simulink model "MPC_implemented_constrained"  (R2023b)
settings: Solver=VariableStepAuto  StartTime=0.0  StopTime=15  RelTol=1e-3
values from neighbouring files (symbols this model uses):
  E = F    [constr_matrix.m]
  F = [F , F1]    [constr_matrix.m]
  FF = F    [constr_matrix.m]
  G = [G , G1]    [constr_matrix.m]
  Gamma = CZ*Gamma    [constr_matrix.m]    (also in mpc_without_constr.m)
  Psi = CZ*Psi    [constr_matrix.m]    (also in mpc_without_constr.m)
  Q = kron(eye(Hp),Qi)    [constr_matrix.m]    (also in lqr_obs.m = [10 0 0 0; mpc_without_constr.m)
  R = kron(eye(Hu),Ri)    [constr_matrix.m]    (also in lqr_obs.m = 1; mpc_without_constr.m)
  T = zeros(l*Hp,m)    [constr_matrix.m]    (also in mpc_without_constr.m)
  TH = CZ*TH    [constr_matrix.m]    (also in mpc_without_constr.m)
  ts = 2e-2    (= 0.02)    [script_mpc.m]
  Ts = 0.02    [system_configuration.m]
  u_nom = 0    [system_configuration.m]
  y_nom = [0 0]    [system_configuration.m]
undefined symbols (not defined in the file or in its folder): a_max, Hu, T_regime, Td, Tsalita
libraries: cstblocks x6
settings Model: Creator=aniello  LastModifiedBy=aniello

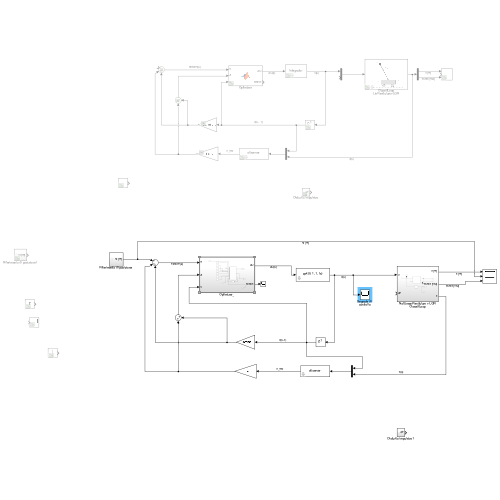
[thumbnail: Simulink's stored preview of the top-level diagram]
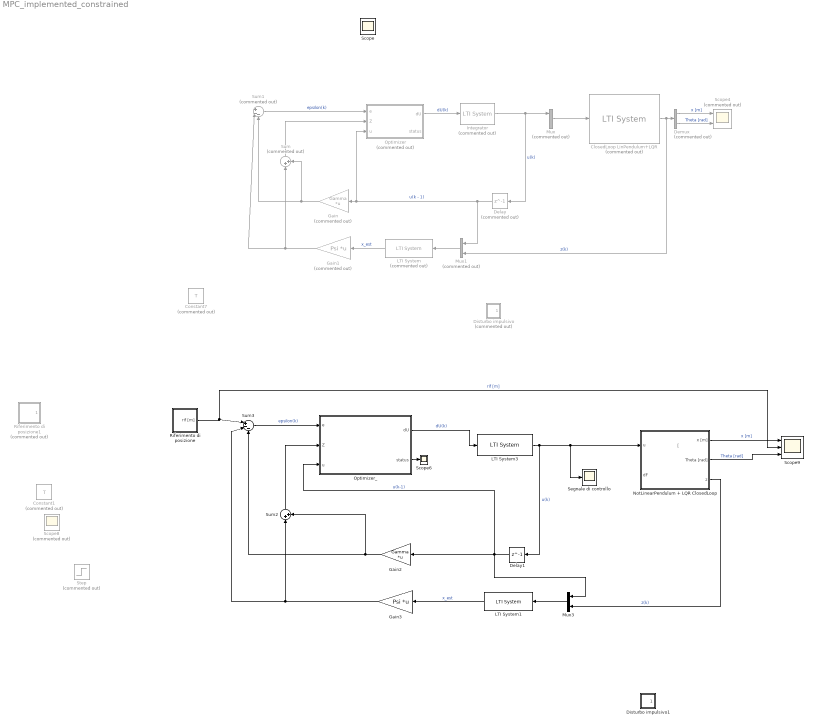
== system MPC_implemented_constrained ==
  note: [
  ClosedLoop LinPendulum+LQR : cstblocks/LTI System  Commented=on  sys=F_k  IC=[]  PadeOrder=0  mask(LTI Block){}
      mask Display: image('pend_im.png');
  Constant1 : Constant  Commented=on  Value=T
  Constant7 : Constant  Commented=on  Value=T
  Delay : Delay  Commented=on  DelayLength=1  SampleTime=ts
  Delay1 : Delay  DelayLength=1  SampleTime=ts
  Demux : Demux  Commented=on  Outputs=2
  Disturbo impulsivo : Subsystem  Commented=on
  Disturbo impulsivo1 : Subsystem
  Gain : Gain  Commented=on  Gain=Gamma  Multiplication=Matrix(K*u)
  Gain1 : Gain  Commented=on  Gain=Psi  Multiplication=Matrix(K*u)
  Gain2 : Gain  Gain=Gamma  Multiplication=Matrix(K*u)
  Gain3 : Gain  Gain=Psi  Multiplication=Matrix(K*u)
  Integrator : cstblocks/LTI System  Commented=on  sys=zpk(0, 1, 1, ts)  IC=[]  PadeOrder=0  mask(LTI Block){}
      mask Display: disp('Integrator');
  LTI System : cstblocks/LTI System  Commented=on  sys=observer  IC=[]  PadeOrder=0
  LTI System1 : cstblocks/LTI System  sys=observer  IC=[]  PadeOrder=0
  LTI System3 : cstblocks/LTI System  sys=zpk(0, 1, 1, ts)  IC=[]  PadeOrder=0
  Mux : Mux  Commented=on  Inputs=2
  Mux1 : Mux  Commented=on  Inputs=2
  Mux3 : Mux  Inputs=2
  NotLinearPendulum + LQR ClosedLoop : Subsystem
  Optimizer : Subsystem  Commented=on
  Optimizer_ : Subsystem
  Riferimento di posizione : Subsystem
  Riferimento di posizione1 : Subsystem  Commented=on
  Scope4 : Scope  Commented=on  NumInputPorts=3
  Scope6 : Scope
  Scope8 : Scope  Commented=on
  Scope9 : Scope  NumInputPorts=3
  Segnale di controllo : Scope
  Step : Step  Commented=on  SampleTime=0
  Sum : Sum  Commented=on  Inputs=|++
  Sum1 : Sum  Commented=on  Inputs=|+--
  Sum2 : Sum  Inputs=|++
  Sum3 : Sum  Inputs=|+--
  Scope : Scope
  wires:
  Mux1/1 -> LTI System/1
  Integrator/1 -> Delay/1, Mux/1  "u(k)"
  Demux/1 -> Scope4/1  "x [m]"
  Demux/2 -> Scope4/3  "Theta [rad]"
  LTI System/1 -> Gain1/1  "x_est"
  Delay/1 -> Gain/1, Optimizer/3(u), Mux1/1  "u(k - 1)"
  Gain/1 -> Sum/2, Sum1/3
  Gain1/1 -> Sum1/2, Sum/1
  Optimizer/1(dU) -> Integrator/1  "dU(k)"
  Sum1/1 -> Optimizer/1(e)  "epsilon(k)"
  Sum/1 -> Optimizer/2(Z)
  Sum3/1 -> Optimizer_/1(e)  "epsilon(k)"
  LTI System1/1 -> Gain3/1  "x_est"
  Delay1/1 -> Optimizer_/3(u), Mux3/1, Gain2/1  "u(k-1)"
  Sum2/1 -> Optimizer_/2(Z)
  Mux3/1 -> LTI System1/1
  Optimizer_/1(dU) -> LTI System3/1  "dU(k)"
  Optimizer_/2(status) -> Scope6/1
  Gain2/1 -> Sum2/2, Sum3/3
  LTI System3/1 -> NotLinearPendulum + LQR ClosedLoop/1(u), Segnale di controllo/1, Delay1/1  "u(k)"
  Gain3/1 -> Sum3/2, Sum2/1
  Mux/1 -> ClosedLoop LinPendulum+LQR/1
  ClosedLoop LinPendulum+LQR/1 -> Mux1/2, Demux/1  "z(k)"
  NotLinearPendulum + LQR ClosedLoop/3(z) -> Mux3/2  "z(k)"
  NotLinearPendulum + LQR ClosedLoop/1(x [m]) -> Scope9/1  "x [m]"
  NotLinearPendulum + LQR ClosedLoop/2(Theta [rad]) -> Scope9/3  "Theta [rad]"
  Riferimento di posizione/1(rif [m]) -> Scope9/2, Sum3/1  "rif [m]"

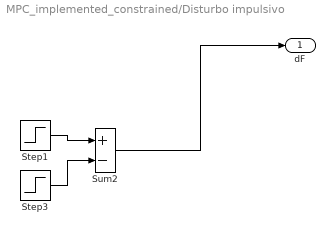
== system MPC_implemented_constrained/Disturbo impulsivo ==
  Step1 : Step  Time=5  After=2  SampleTime=0
  Step3 : Step  Time=5.04  After=2  SampleTime=0
  Sum2 : Sum  Inputs=+-
  dF : Outport
  wires:
  Sum2/1 -> dF/1
  Step3/1 -> Sum2/2
  Step1/1 -> Sum2/1

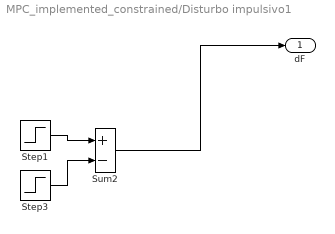
== system MPC_implemented_constrained/Disturbo impulsivo1 ==
  Step1 : Step  Time=5  After=2  SampleTime=0
  Step3 : Step  Time=5.04  After=2  SampleTime=0
  Sum2 : Sum  Inputs=+-
  dF : Outport
  wires:
  Sum2/1 -> dF/1
  Step3/1 -> Sum2/2
  Step1/1 -> Sum2/1

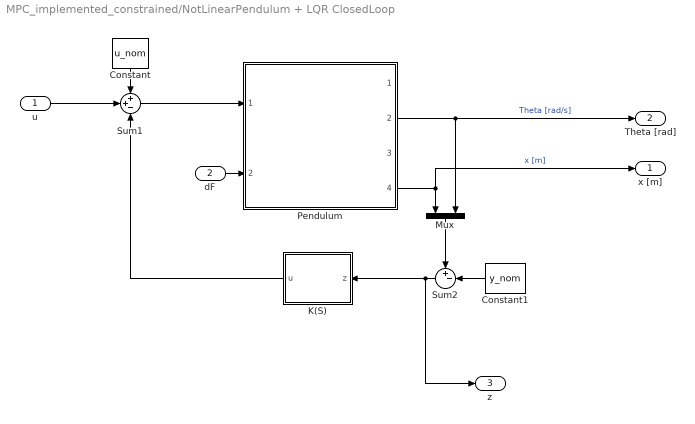
== system MPC_implemented_constrained/NotLinearPendulum + LQR ClosedLoop ==
  u : Inport
  dF : Inport  Port=2
  Constant : Constant  Value=u_nom
  Constant1 : Constant  Value=y_nom
  K(S) : Subsystem
  Mux : Mux  Inputs=2
  Pendulum : Subsystem  ReferencedSubsystem=pendulum
  Sum1 : Sum  Inputs=++-
  Sum2 : Sum  Inputs=+-|
  x [m] : Outport
  Theta [rad] : Outport  Port=2
  z : Outport  Port=3
  wires:
  dF/1 -> Pendulum/2
  Constant1/1 -> Sum2/2
  K(S)/1(u) -> Sum1/3
  Sum1/1 -> Pendulum/1
  Mux/1 -> Sum2/1
  Pendulum/2 -> Theta [rad]/1, Mux/2  "Theta [rad/s]"
  u/1 -> Sum1/2
  Constant/1 -> Sum1/1
  Sum2/1 -> z/1, K(S)/1(z)
  Pendulum/4 -> x [m]/1, Mux/1  "x [m]"

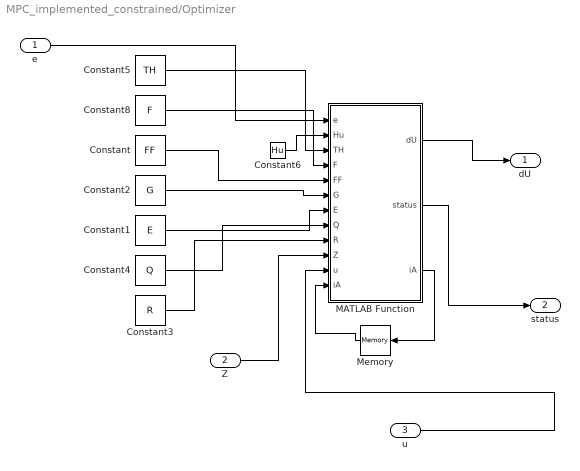
== system MPC_implemented_constrained/Optimizer ==
  e : Inport
  Z : Inport  Port=2
  u : Inport  Port=3
  Constant : Constant  Value=FF  VectorParams1D=off  OutDataTypeStr=double
  Constant1 : Constant  Value=E  OutDataTypeStr=double
  Constant2 : Constant  Value=G  OutDataTypeStr=double
  Constant3 : Constant  Value=R  OutDataTypeStr=double
  Constant4 : Constant  Value=Q  OutDataTypeStr=double
  Constant5 : Constant  Value=TH  OutDataTypeStr=double
  Constant6 : Constant  Value=Hu  VectorParams1D=off
  Constant8 : Constant  Value=F  VectorParams1D=off  OutDataTypeStr=double
  MATLAB Function : MATLAB Function  TreatAsAtomicUnit=on
  Memory : Memory  InitialCondition=false(360,1)
  dU : Outport
  status : Outport  Port=2
  wires:
  MATLAB Function/2(status) -> status/1
  Z/1 -> MATLAB Function/10(Z)
  MATLAB Function/1(dU) -> dU/1
  Constant6/1 -> MATLAB Function/2(Hu)
  Constant8/1 -> MATLAB Function/4(F)
  Constant1/1 -> MATLAB Function/7(E)
  Constant/1 -> MATLAB Function/5(FF)
  Constant4/1 -> MATLAB Function/8(Q)
  e/1 -> MATLAB Function/1(e)
  Memory/1 -> MATLAB Function/12("iA ")
  u/1 -> MATLAB Function/11(u)
  MATLAB Function/3(iA) -> Memory/1
  Constant5/1 -> MATLAB Function/3(TH)
  Constant3/1 -> MATLAB Function/9(R)
  Constant2/1 -> MATLAB Function/6(G)

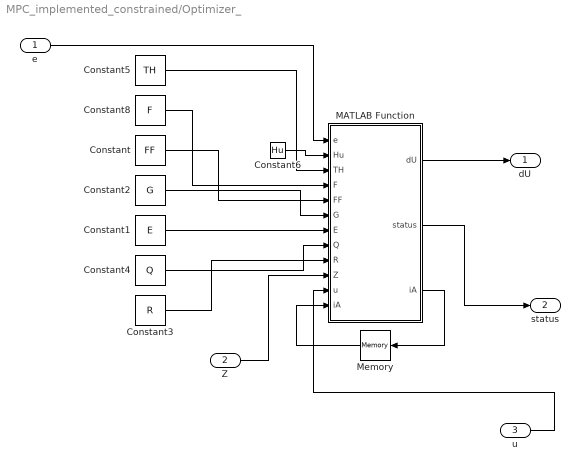
== system MPC_implemented_constrained/Optimizer_ ==
  e : Inport
  Z : Inport  Port=2
  u : Inport  Port=3
  Constant : Constant  Value=FF  VectorParams1D=off  OutDataTypeStr=double
  Constant1 : Constant  Value=E  OutDataTypeStr=double
  Constant2 : Constant  Value=G  OutDataTypeStr=double
  Constant3 : Constant  Value=R  OutDataTypeStr=double
  Constant4 : Constant  Value=Q  OutDataTypeStr=double
  Constant5 : Constant  Value=TH  OutDataTypeStr=double
  Constant6 : Constant  Value=Hu  VectorParams1D=off
  Constant8 : Constant  Value=F  VectorParams1D=off  OutDataTypeStr=double
  MATLAB Function : MATLAB Function  TreatAsAtomicUnit=on
  Memory : Memory  InitialCondition=false(360,1)
  dU : Outport
  status : Outport  Port=2
  wires:
  MATLAB Function/2(status) -> status/1
  Z/1 -> MATLAB Function/10(Z)
  MATLAB Function/1(dU) -> dU/1
  Constant6/1 -> MATLAB Function/2(Hu)
  Constant8/1 -> MATLAB Function/4(F)
  Constant1/1 -> MATLAB Function/7(E)
  Constant/1 -> MATLAB Function/5(FF)
  Constant4/1 -> MATLAB Function/8(Q)
  e/1 -> MATLAB Function/1(e)
  Memory/1 -> MATLAB Function/12("iA ")
  u/1 -> MATLAB Function/11(u)
  MATLAB Function/3(iA) -> Memory/1
  Constant5/1 -> MATLAB Function/3(TH)
  Constant3/1 -> MATLAB Function/9(R)
  Constant2/1 -> MATLAB Function/6(G)

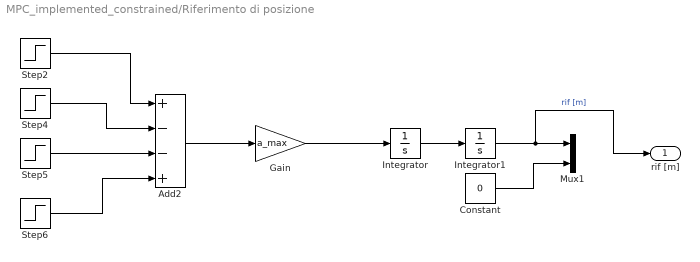
== system MPC_implemented_constrained/Riferimento di posizione ==
  Add2 : Sum  Inputs=+--+
  Constant : Constant  Value=0
  Gain : Gain  Gain=a_max
  Integrator : Integrator
  Integrator1 : Integrator
  Mux1 : Mux  Inputs=2
  Step2 : Step  SampleTime=0
  Step4 : Step  Time=Tsalita+1  SampleTime=0
  Step5 : Step  Time=Tsalita+T_regime+1  SampleTime=0
  Step6 : Step  Time=Tsalita+T_regime+Td+1  SampleTime=0
  rif [m] : Outport
  wires:
  Step6/1 -> Add2/4
  Step5/1 -> Add2/3
  Gain/1 -> Integrator/1
  Integrator/1 -> Integrator1/1
  Add2/1 -> Gain/1
  Step2/1 -> Add2/1
  Step4/1 -> Add2/2
  Constant/1 -> Mux1/2
  Integrator1/1 -> rif [m]/1, Mux1/1  "rif [m]"

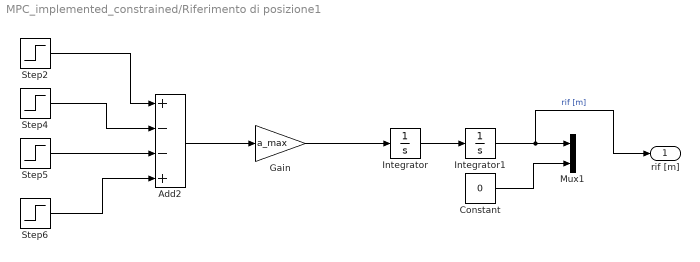
== system MPC_implemented_constrained/Riferimento di posizione1 ==
  Add2 : Sum  Inputs=+--+
  Constant : Constant  Value=0
  Gain : Gain  Gain=a_max
  Integrator : Integrator
  Integrator1 : Integrator
  Mux1 : Mux  Inputs=2
  Step2 : Step  SampleTime=0
  Step4 : Step  Time=Ts+1  SampleTime=0
  Step5 : Step  Time=Ts+T_regime+1  SampleTime=0
  Step6 : Step  Time=Ts+T_regime+Td+1  SampleTime=0
  rif [m] : Outport
  wires:
  Integrator1/1 -> Mux1/1, rif [m]/1  "rif [m]"
  Constant/1 -> Mux1/2
  Step4/1 -> Add2/2
  Step2/1 -> Add2/1
  Add2/1 -> Gain/1
  Integrator/1 -> Integrator1/1
  Gain/1 -> Integrator/1
  Step5/1 -> Add2/3
  Step6/1 -> Add2/4

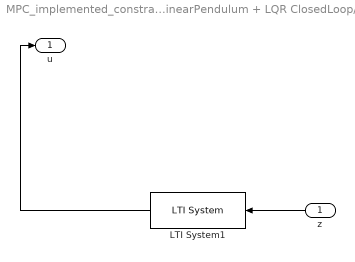
== system MPC_implemented_constrained/NotLinearPendulum + LQR ClosedLoop/K(S) ==
  z : Inport
  LTI System1 : cstblocks/LTI System  sys=K_s  IC=[]  PadeOrder=0
  u : Outport
  wires:
  LTI System1/1 -> u/1
  z/1 -> LTI System1/1

== matlab function MPC_implemented_constrained/Optimizer_/MATLAB Function ==
  data: e input; Hu input; TH input; F input; FF input; G input; E input; Q input; R input; Z input; dU output; u input; iA input boolean; status output; iA output
function [dU,status,iA]  = fnc(e, Hu, TH, F,FF, G, E, Q, R, Z, u, iA) %#codegen

[dU,status,iA] = MPC_constr(e, Hu, TH, F,FF, G, E, Q, R, Z, u, iA);

end

== matlab function MPC_implemented_constrained/Optimizer/MATLAB Function ==
  data: e input; Hu input; TH input; F input; FF input; G input; E input; Q input; R input; Z input; dU output; u input; iA input boolean; status output; iA output
function [dU,status,iA]  = fnc(e, Hu, TH, F,FF, G, E, Q, R, Z, u, iA) %#codegen

[dU,status,iA] = MPC_constr(e, Hu, TH, F,FF, G, E, Q, R, Z, u, iA);

end
